simulink model "CellVoltageDiagnostics_slrt"  (R2022a)
settings: configuration reference "BMS_Sw_CodeGenConfigSLRT" (kept outside this file)
undefined symbols (not defined in the file): MaxDeltaCellVoltage, OverCellVoltageLimit, UnderCellVoltageLimit
settings Model: DataDictionary=CellVoltageDiagnostics_DD.sldd  EnableAccessToBaseWorkspace=off  ExtModeTrigDuration=5  Creator=Chirag Patel  LastModifiedBy=timo.straessle
settings ConfigSetRef: SourceName=BMS_Sw_CodeGenConfigSLRT

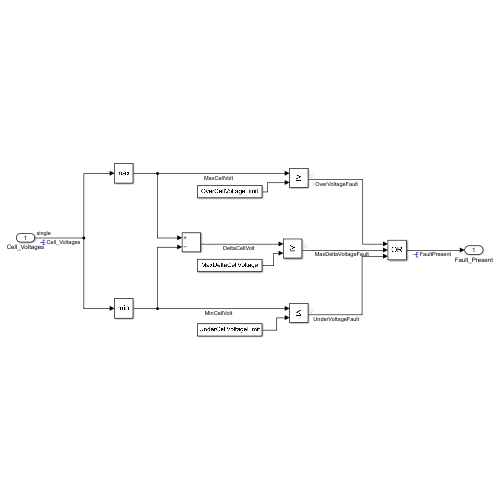
[thumbnail: Simulink's stored preview of the top-level diagram]
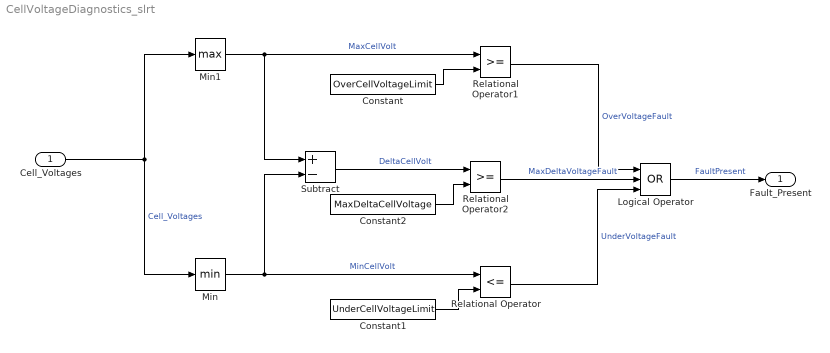
== system CellVoltageDiagnostics_slrt ==
  Cell_Voltages : Inport  OutDataTypeStr=single  PortDimensions=6  SampleTime=[0.10000000000000001,0]
  Constant : Constant  Value=OverCellVoltageLimit
  Constant1 : Constant  Value=UnderCellVoltageLimit
  Constant2 : Constant  Value=MaxDeltaCellVoltage
  Logical Operator : Logic  Operator=OR  Inputs=3  AllPortsSameDT=off  OutDataTypeStr=boolean
  Min : MinMax
  Min1 : MinMax  Function=max
  Relational Operator : RelationalOperator  Operator=<=  OutDataTypeStr=boolean  RndMeth=Simplest  InputSameDT=off
  Relational Operator1 : RelationalOperator  OutDataTypeStr=boolean  RndMeth=Simplest  InputSameDT=off
  Relational Operator2 : RelationalOperator  OutDataTypeStr=boolean  RndMeth=Simplest  InputSameDT=off
  Subtract : Sum  Inputs=+-
  Fault_Present : Outport  VectorParamsAs1DForOutWhenUnconnected=off
  wires:
  Cell_Voltages/1 -> Min1/1, Min/1  "Cell_Voltages"
  Logical Operator/1 -> Fault_Present/1  "FaultPresent"
  Min1/1 -> Subtract/1, Relational Operator1/1  "MaxCellVolt"
  Min/1 -> Subtract/2, Relational Operator/1  "MinCellVolt"
  Constant1/1 -> Relational Operator/2
  Constant/1 -> Relational Operator1/2
  Subtract/1 -> Relational Operator2/1  "DeltaCellVolt"
  Constant2/1 -> Relational Operator2/2
  Relational Operator2/1 -> Logical Operator/2  "MaxDeltaVoltageFault"
  Relational Operator1/1 -> Logical Operator/1  "OverVoltageFault"
  Relational Operator/1 -> Logical Operator/3  "UnderVoltageFault"
